simulink model "EXAMPLE"  (Simulink 6.6)
settings: Solver=ode45  StartTime=0.0  StopTime=10.0  RelTol=1e-3
settings Model: Creator=cebolletas  LastModifiedBy=cebolletas

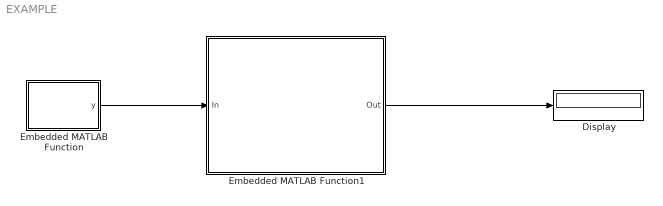
== system EXAMPLE ==
  Display : Display
  Embedded MATLAB Function : Stateflow chart
  Embedded MATLAB Function1 : Stateflow chart
  wires:
  Embedded MATLAB Function1/1(Out) -> Display/1
  Embedded MATLAB Function/1(y) -> Embedded MATLAB Function1/1(In)

== matlab function Embedded MATLAB Function1 ==
  data: In input inherited; Out output inherited
function Out = hexsingle2num(In)

%*************************************************************************
% Block hexsingle2num
% Created in Simulink r2007a
%
% Author: Daniel Martin Martin
% email: daniel.martin@savant-eyd.com
%
% SAVANT ENERGÍA Y DINÁMICA
% www.savant-eyd.com
% 
% October 2008
%
%*************************************************************************
% This block converts the 32 bits hex input into the corresponding FLOAT,
% using the IEEE 32 bits float format. 
%*************************************************************************


%*************************************************************************
% This block is based on the Matlab function hexsingle2num.m created by
% Mark Lubinski, which is based on the standard hex2num Matlab function.
% Check out Mark's function at:
% http://www.mathworks.com/matlabcentral/fileexchange/loadFile.do?objectId=6927&objectType=FILE
%*************************************************************************


%*************************************************************************
% WARNING WARNING WARNING WARNING WARNING WARNING WARNING WARNING WARNING
%*************************************************************************
% Hex numbers are treated as strings in Matlab and Simulink. Any Simulink
% block can only have numerical input or output so the 32 bits hex imput 
% needs to be converted into a number before sending it to this block. 
% This have to be done with the hex2num() function. This function will 
% trasnform our hex number into an integer, so it WONT be the desired 
% final number, but it will be fine for sending it to this block.
%*************************************************************************
% So it is NECESSARY to use hex2num() on the previous block output before
% conecting it to this block.
%*************************************************************************
%In the ZIP file there is an example of the usage, so PLEASE check it out.
%*************************************************************************


%*************************************************************************
% WARNING WARNING WARNING WARNING WARNING WARNING WARNING WARNING WARNING
%*************************************************************************
%During Execution Simulink will show you warnings messages. IGNORE THEM.
%*************************************************************************







%*************************************************************************
% We set all the variables that we are going to use (mandatory in Simulink)
%*************************************************************************

a='papapapapapapapa';
aux3=0;
aux4=0;
neg=0;
t=0;


%*************************************************************************
% We undo the input change, to get the 32 bits hex number.
%*************************************************************************

a=num2hex(In);
s=a(1:8);

%*************************************************************************
%*************************************************************************
[row,col] = size(s);
d = zeros(row,8);
x = zeros(row,1);
blanks = find(s==' '); % Find the blanks at the end
s=lower(s);


%*************************************************************************
%*************************************************************************
for i=1:8
   switch(s(i))
       case '0' 
           d(i)=0;
       case '1' 
           d(i)=1;
       case '2' 
           d(i)=2;
       case '3' 
           d(i)=3;
       case '4' 
           d(i)=4;
       case '5' 
           d(i)=5;
       case '6' 
           d(i)=6;
       case '7' 
           d(i)=7;
       case '8' 
           d(i)=8;
       case '9' 
           d(i)=9;
       case 'a' 
           d(i)=10;
       case 'b' 
           d(i)=11;
       case 'c' 
           d(i)=12;
       case 'd' 
           d(i)=13;
       case 'e' 
           d(i)=14;           
       case 'f' 
           d(i)=15;
   end
    
end


if (d(1) > 7)
    neg = 1;
end
d(1) = d(1)-8*neg;

%*************************************************************************
%*************************************************************************


expBit = (d(:,3) > 7);
e = 32*d(:,1) + 2*d(:,2) + expBit - 127;
d(:,3) = d(:,3)-8*expBit;  


sixteens = [16;256;4096;65536;1048576;16777216];
multiplier = 2./[sixteens];
f = d(:,3:8)*multiplier;

%*************************************************************************
%*************************************************************************

% Scale the fraction by 2 to the exponent.
overinf = find((e>127) & (f==0));
if ~isempty(overinf)
    aux=overinf;
    %x(aux) = inf; 
end

overNaN = find((e>127) & (f~=0));
if ~isempty(overNaN)
    aux=overNaN;
    %x(aux) = NaN; 
end

underflow = find(e<-126);
if ~isempty(underflow) 
    %x(underflow) = pow2(f(underflow),-126); 
end


allothers = find((e<=127) & (e>=-126));
if ~isempty(allothers)
    
    aux3=1+f;
    aux4=e;
    x = pow2(aux3,aux4); 
end

negatives = find(neg==1);
if ~isempty(negatives)
    x = -x; 
end

Out=x;

%*************************************************************************
% End of the function.
%*************************************************************************

== matlab function Embedded MATLAB Function ==
  data: y output inherited
function y = fcn()

y=0;

hexnumber='42b40000';


y = hex2num(hexnumber);
